simulink model "Vehicle_suspension"  (R2020b)
settings: Solver=VariableStepAuto  StartTime=0.0  StopTime=10.0  RelTol=1e-3
settings Model: Creator=sayali  LastModifiedBy=sayali

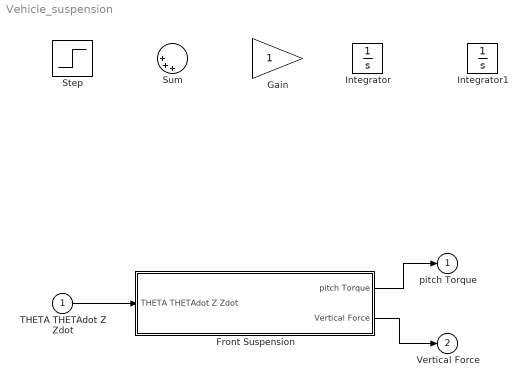
== system Vehicle_suspension ==
  THETA THETAdot Z Zdot : Inport
  Front Suspension : Subsystem
  Gain : Gain
  Integrator : Integrator
  Integrator1 : Integrator
  Step : Step  SampleTime=0
  Sum : Sum  Inputs=||+++
  pitch Torque : Outport  VectorParamsAs1DForOutWhenUnconnected=off
  Vertical Force : Outport  Port=2  VectorParamsAs1DForOutWhenUnconnected=off
  wires:
  THETA THETAdot Z Zdot/1 -> Front Suspension/1(THETA THETAdot Z Zdot)
  Front Suspension/1(pitch Torque) -> pitch Torque/1
  Front Suspension/2(Vertical Force) -> Vertical Force/1

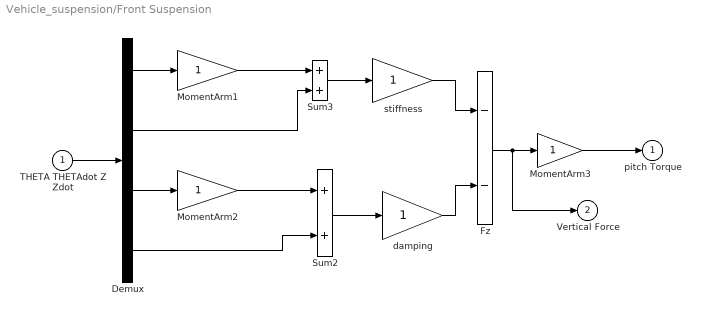
== system Vehicle_suspension/Front Suspension ==
  THETA THETAdot Z Zdot : Inport
  Demux : Demux
      settings: DisplayOption=none
  Fz : Sum  Inputs=--  InputSameDT=on  SaturateOnIntegerOverflow=on  OutDataTypeStr=Inherit: Same as first input
  MomentArm1 : Gain  SaturateOnIntegerOverflow=on  OutDataTypeStr=Inherit: Same as input  ParamDataTypeStr=Inherit: Same as input
  MomentArm2 : Gain  SaturateOnIntegerOverflow=on  OutDataTypeStr=Inherit: Same as input  ParamDataTypeStr=Inherit: Same as input
  MomentArm3 : Gain  SaturateOnIntegerOverflow=on  OutDataTypeStr=Inherit: Same as input  ParamDataTypeStr=Inherit: Same as input
  Sum2 : Sum  InputSameDT=on  SaturateOnIntegerOverflow=on  OutDataTypeStr=Inherit: Same as first input
  Sum3 : Sum  InputSameDT=on  SaturateOnIntegerOverflow=on  OutDataTypeStr=Inherit: Same as first input
  damping : Gain  SaturateOnIntegerOverflow=on  OutDataTypeStr=Inherit: Same as input  ParamDataTypeStr=Inherit: Same as input
  stiffness : Gain  SaturateOnIntegerOverflow=on  OutDataTypeStr=Inherit: Same as input  ParamDataTypeStr=Inherit: Same as input
  pitch Torque : Outport  VectorParamsAs1DForOutWhenUnconnected=off
  Vertical Force : Outport  Port=2  VectorParamsAs1DForOutWhenUnconnected=off
  wires:
  Demux/1 -> MomentArm1/1
  Sum3/1 -> stiffness/1
  THETA THETAdot Z Zdot/1 -> Demux/1
  Fz/1 -> Vertical Force/1, MomentArm3/1
  stiffness/1 -> Fz/1
  damping/1 -> Fz/2
  MomentArm1/1 -> Sum3/1
  MomentArm3/1 -> pitch Torque/1
  MomentArm2/1 -> Sum2/1
  Demux/4 -> Sum2/2
  Sum2/1 -> damping/1
  Demux/2 -> Sum3/2
  Demux/3 -> MomentArm2/1
